simulink model "CameraMotion"  (Simulink 4.00)
settings: Solver=ode45  StartTime=0.0  StopTime=10.0  RelTol=1e-3
libraries: vs x2
settings Model: LastModifiedBy=ecervera

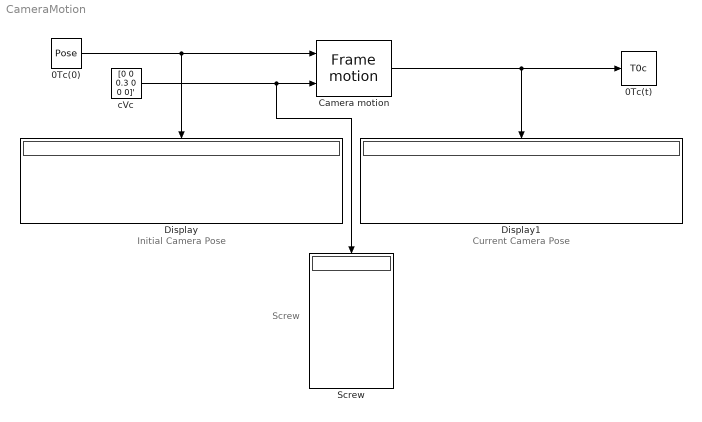
== system CameraMotion ==
  note: Initial Camera Pose
  note: Current Camera Pose
  note: Screw
  0Tc(0) : vs/Pose/Pose  x=0  y=0  z=-1.5  r=RPY  phi=0  theta=0  psi=0
  0Tc(t) : ToWorkspace  VariableName=T0c  SampleTime=-1  SaveFormat=StructureWithTime
  Camera motion : vs/Pose/Frame motion
      settings: RTWFcnNameOpts=Auto  RTWFileNameOpts=Auto
  Display : Display
      settings: Orientation=down  Format=short
  Display1 : Display
      settings: Orientation=down  Format=short
  "Screw " : Display
      settings: Orientation=down  Format=short
  cVc : Constant  Value=[0 0 0.3 0 0 0]'  VectorParams1D=off
  wires:
  0Tc(0)/1 -> Camera motion/1, Display/1
  Camera motion/1 -> Display1/1, 0Tc(t)/1
  cVc/1 -> Camera motion/2, "Screw "/1
